simulink model "advance_compensator_simulink"  (R2016a)
settings: Solver=VariableStepAuto  StartTime=0.0  StopTime=10.0  RelTol=1e-3
values from neighbouring files (symbols this model uses):
  Kc = Kp_desejado/Kp_antigo    (= 99)    [adv_lag_igual.m]    (also in advance_and_lagging_compensator.m = (1)/abs(((s1+zero_adv)/(s1+polo_adv))*planta); advance_compensator.m = (1)/abs(((s1+zero_cont1)/(s1+polo_cont1))*planta); lagging_compensator.m = (1)/abs(((s1+zero_lag)/(s1+polo_lag))*planta))
  polo_cont1 = 5.75    [advance_compensator.m]
  zero_cont1 = 3.87    [advance_compensator.m]
settings Model: Creator=jessa  LastModifiedBy=jessa

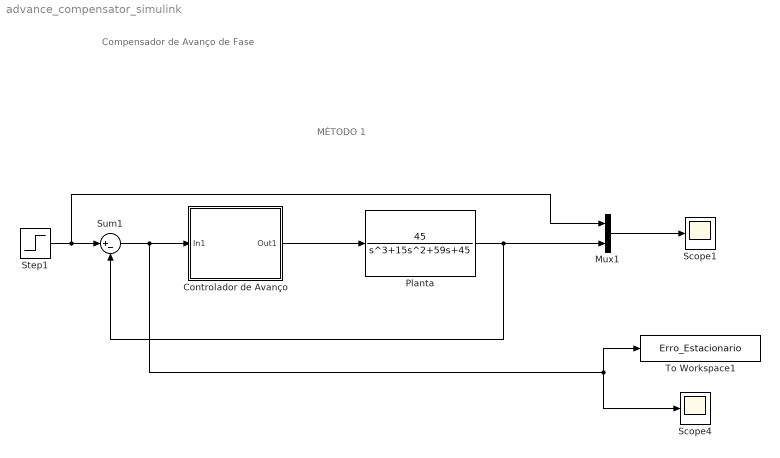
== system advance_compensator_simulink ==
  note: Compensador de Avanço de Fase
  note: MÉTODO 1
  Controlador de Avanço : Subsystem
  Mux1 : Mux  Inputs=2
  Planta : TransferFcn  Numerator=[45]  Denominator=[1 15 59 45]
  Scope1 : Scope
  Scope4 : Scope
  Step1 : Step  Time=0  SampleTime=0
  Sum1 : Sum  Inputs=|+-
  To Workspace1 : ToWorkspace  VariableName=Erro_Estacionario  SampleTime=-1
  wires:
  Mux1/1 -> Scope1/1
  Planta/1 -> Sum1/2, Mux1/2
  Step1/1 -> Sum1/1, Mux1/1
  Controlador de Avanço/1(Out1) -> Planta/1
  Sum1/1 -> To Workspace1/1, Scope4/1, Controlador de Avanço/1(In1)

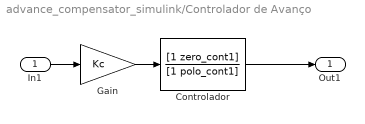
== system advance_compensator_simulink/Controlador de Avanço ==
  In1 : Inport
  Controlador : TransferFcn  Numerator=[1 zero_cont1]  Denominator=[1 polo_cont1]
  Gain : Gain  Gain=Kc
  Out1 : Outport
  wires:
  In1/1 -> Gain/1
  Gain/1 -> Controlador/1
  Controlador/1 -> Out1/1
